simulink model "Super5"  (Simulink 5.0)
settings: Solver=ode45  StartTime=0.0  StopTime=10.0  RelTol=1e-3
settings Model: Creator=scaife  LastModifiedBy=scaife  ExtModeAutoUpdateStatusClock=off

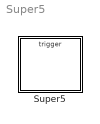
== system Super5 ==
  Super5 : Stateflow chart

== stateflow chart Super5 ==
  state A
    state A1
    (default) -> A1
  state B
    state B1
    (default) -> B1
  state D
    state D1
    (default) -> D1
  state C
    state C1
    (default) -> C1
  D1 -> A1 : E
  A1 -> B1 : E
  B1 -> A1 : F
  B1 -> C1 : E
  C1 -> D1 : E
  A -> B : G
  B -> A : H
  A1 -> D1 : F
  C1 -> B1 : F
  D1 -> C1 : F
  A -> D : H
  D -> A : G
  D -> C : H
  C -> D : G
  C -> B : H
  B -> C : G
  (default) -> A
  events: E input EITHER_EDGE_EVENT; G input EITHER_EDGE_EVENT; F input EITHER_EDGE_EVENT; H input EITHER_EDGE_EVENT
